simulink model "Example_2"  (R2020b)
settings: Solver=VariableStepAuto  StartTime=0.0  StopTime=0.01  RelTol=1e-3
libraries: fl_lib x15, nesl_utility x4, ee_lib x1
settings Model: Creator=zaliyazici  LastModifiedBy=zaliyazici

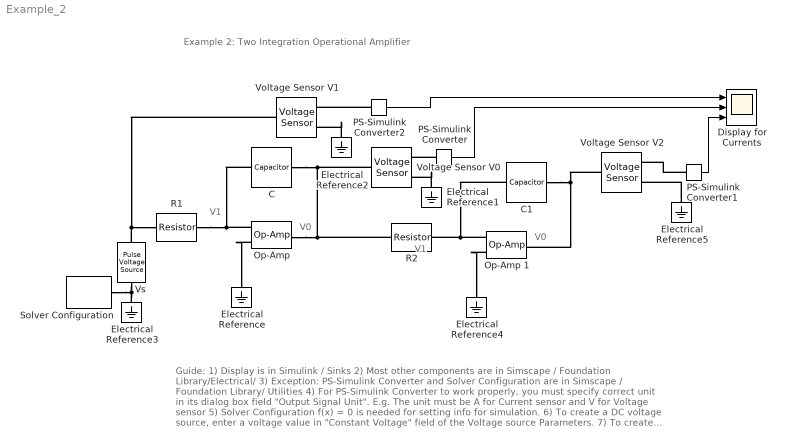
== system Example_2 ==
  note: V0
  note: Guide:
      | 1) Display is in Simulink / Sinks
      | 2) Most other components are in Simscape / Foundation Library/Electrical/
      | 3) Exception: PS-Simulink Converter and Solver Configuration are in Simscape / Foundation Library/ Utilities
      | 4) For PS-Simulink Converter to work properly, you must specify correct unit in its dialog box field "Output Signal Unit".
      | E.g. The unit must be A for Current sensor and V for Voltage sensor
      | 5) Solver Configuration f(x) = 0 is needed for setting info for simulation.
      | 6) To create a DC voltage source, enter a voltage value in "Constant Voltage" field of the Voltage source Parameters.
      | 7) To create "Annotation", double-click a location on project page and select "Create annotation" from the prompt. Then, type any text you want to clarify your circuit. E.g. "Display for Current".
      | 8) To understand how to use a component, right-click on the component and select "Help".
      | Measurement: Node voltages V1, and V0
  note: Example 2: Two Integration Operational Amplifier
  note: V1
  note: V0
  note: V1
  C : fl_lib/Electrical/Electrical Elements/Capacitor  c=100 nF  r=1e-6 Ohm  g=0 1/Ohm  i_specify=off  i_priority=None  i=0 A  i_nominal_specify=off  i_nominal_unit=A  i_nominal_value=1  v_specify=off  v_priority=None  v=0 V  v_nominal_specify=off  v_nominal_unit=V  v_nominal_value=1  vc_specify=off  vc_priority=High  vc=0 V  vc_nominal_specify=off  vc_nominal_unit=V  vc_nominal_value=1
      settings: AttributesFormatString=%<c> %<c_unit>
  C1 : fl_lib/Electrical/Electrical Elements/Capacitor  c=100 nF  r=1e-6 Ohm  g=0 1/Ohm  i_specify=off  i_priority=None  i=0 A  i_nominal_specify=off  i_nominal_unit=A  i_nominal_value=1  v_specify=off  v_priority=None  v=0 V  v_nominal_specify=off  v_nominal_unit=V  v_nominal_value=1  vc_specify=off  vc_priority=High  vc=0 V  vc_nominal_specify=off  vc_nominal_unit=V  vc_nominal_value=1
      settings: AttributesFormatString=%<c> %<c_unit>
  Display for Currents : Scope  NumInputPorts=3
  Electrical Reference{,1..5} (6 alike) : fl_lib/Electrical/Electrical Elements/Electrical Reference
  "Op-Amp " : fl_lib/Electrical/Electrical Elements/Op-Amp  outI_specify=off  outI_priority=None  outI=0 A  outI_nominal_specify=off  outI_nominal_unit=A  outI_nominal_value=1
  Op-Amp 1 : fl_lib/Electrical/Electrical Elements/Op-Amp  outI_specify=off  outI_priority=None  outI=0 A  outI_nominal_specify=off  outI_nominal_unit=A  outI_nominal_value=1
  PS-Simulink Converter : nesl_utility/PS-Simulink Converter  PhysicalDomain=network_engine_domain  SubClassName=ps_output  LeftPortType=input  RightPortType=output  PseudoPeriodic=off  Frequencies=[]  Unit=V  AffineConversion=off
  PS-Simulink Converter1 : nesl_utility/PS-Simulink Converter  PhysicalDomain=network_engine_domain  SubClassName=ps_output  LeftPortType=input  RightPortType=output  PseudoPeriodic=off  Frequencies=[]  Unit=V  AffineConversion=off
  PS-Simulink Converter2 : nesl_utility/PS-Simulink Converter  PhysicalDomain=network_engine_domain  SubClassName=ps_output  LeftPortType=input  RightPortType=output  PseudoPeriodic=off  Frequencies=[]  Unit=V  AffineConversion=off
  R1 : fl_lib/Electrical/Electrical Elements/Resistor  R=2 kOhm  i_specify=off  i_priority=None  i=0 A  i_nominal_specify=off  i_nominal_unit=A  i_nominal_value=1  v_specify=off  v_priority=None  v=0 V  v_nominal_specify=off  v_nominal_unit=V  v_nominal_value=1
      settings: AttributesFormatString=%<R> %<R_unit>  LogSimulationData=on
  R2 : fl_lib/Electrical/Electrical Elements/Resistor  R=2 kOhm  i_specify=off  i_priority=None  i=0 A  i_nominal_specify=off  i_nominal_unit=A  i_nominal_value=1  v_specify=off  v_priority=None  v=0 V  v_nominal_specify=off  v_nominal_unit=V  v_nominal_value=1
      settings: AttributesFormatString=%<R> %<R_unit>  LogSimulationData=on
  Solver Configuration : nesl_utility/Solver Configuration  PhysicalDomain=network_engine_domain  SubClassName=solver  LeftPortType=input  RightPortType=generic  Tones=[]  Harmonics=[]  SimulateNoise=off  Profile=off  UseLocalSampling=off  EnableSwitchedLinearOptims=on  FrequencyDomain=off  UseCCode=off  RelTol=0.001  AbsTol=1e-06  MinStep=1e-09  ToWorkspace=off  RevertToSquareIcSolve=off  NumHomotopyIterations=100  PhasorMode=off  PhasorModeNumHarmonics=1  DoDC=off  ResidualTolerance=1e-09  UseLocalSolver=off  LocalSolverChoice=NE_BACKWARD_EULER_ADVANCER  LocalSolverSampleTime=0.001  DoFixedCost=off  MaxNonlinIter=3  MaxModeIter=2  ComputeImpulses=off  ImpulseIterations=2  LinearAlgebra=auto  EquationFormulation=NE_TIME_EF  DelaysMemoryBudget=1024  AutomaticFiltering=on  FilteringTimeConstant=0.001  PartitionStorageMethod=AS_NEEDED  PartitionMemoryBudget=1024  PartitionMethod=ROBUST
  Voltage Sensor V0 : fl_lib/Electrical/Electrical Sensors/Voltage Sensor
  Voltage Sensor V1 : fl_lib/Electrical/Electrical Sensors/Voltage Sensor
  Voltage Sensor V2 : fl_lib/Electrical/Electrical Sensors/Voltage Sensor
  Vs : ee_lib/Additional Components/SPICE Sources/Pulse Voltage Source  V1=-1 V  V2=1 V  TD=0 s  TR=1e-9 s  TF=1e-9 s  PW=1 ms  PER=2 ms
      settings: SourceProductBaseCode=PS  InternalSimscapePortConfiguration="{\"Bottom\":[],\"Left\":[{\"id\":\"p\",\"label\":\"\",\"type\":\"foundation.electrical.electrical\"}],\"Right\":[{\"id\":\"n\",\"label\":\"\",\"type\":\"foundation.electrical.electrical\"}],\"Top\":[]}"
  wires:
  PS-Simulink Converter/1 -> Display for Currents/2
  PS-Simulink Converter2/1 -> Display for Currents/1
  PS-Simulink Converter1/1 -> Display for Currents/3
  connections:
  Vs/LConn1 -- Voltage Sensor V1/LConn1 -- R1/LConn1
  "Op-Amp "/LConn1 -- Electrical Reference/LConn1
  Electrical Reference1/LConn1 -- Voltage Sensor V0/RConn2
  PS-Simulink Converter/LConn1 -- Voltage Sensor V0/RConn1
  PS-Simulink Converter2/LConn1 -- Voltage Sensor V1/RConn1
  "Op-Amp "/RConn1 -- C/RConn1 -- Voltage Sensor V0/LConn1 -- R2/LConn1
  Electrical Reference2/LConn1 -- Voltage Sensor V1/RConn2
  Solver Configuration/RConn1 -- Vs/RConn1 -- Electrical Reference3/LConn1
  R1/RConn1 -- C/LConn1 -- "Op-Amp "/LConn2
  Op-Amp 1/LConn2 -- C1/LConn1 -- R2/RConn1
  Op-Amp 1/LConn1 -- Electrical Reference4/LConn1
  C1/RConn1 -- Voltage Sensor V2/LConn1 -- Op-Amp 1/RConn1
  PS-Simulink Converter1/LConn1 -- Voltage Sensor V2/RConn1
  Electrical Reference5/LConn1 -- Voltage Sensor V2/RConn2
